simulink model "VCVS_lin_in_comm_out_comm"  (Simulink 7.5)
settings: Solver=ode45  StartTime=0.0  StopTime=10.0  RelTol=1e-3
settings Model: Creator=tugui_cat  LastModifiedBy=tugui
settings DebuggingCC: StrictBusMsg=Warning

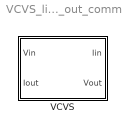
== system VCVS_lin_in_comm_out_comm ==
  VCVS : Subsystem  mask{Num_TF_dir1=1, Den_TF_dir1=1, Num_TF_inv1=1, Den_TF_inv1=1, Num_Zin1=1, Den_Zin1=1, Num_Zout1=1, Den_Zout1=1, OffIn11=0, OffIn12=0, OffOut11=0, OffOut12=0}
      mask help: Current-Controlled-Current-Source - linear model

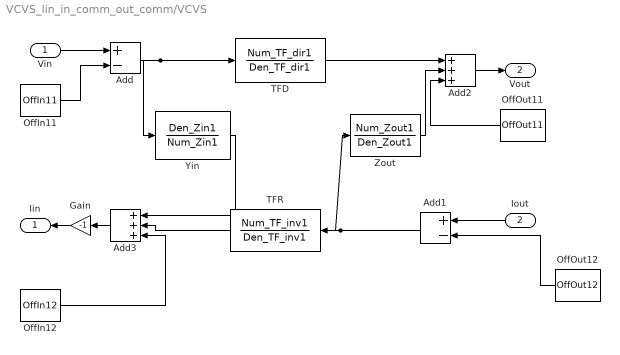
== system VCVS_lin_in_comm_out_comm/VCVS ==
  Vin : Inport
  Iout : Inport  Port=2
  Add : Sum  Inputs=+-  OutDataType=fixdt(1, 16)  OutScaling=2^-10
  Add1 : Sum  Inputs=+-  OutDataType=fixdt(1, 16)  OutScaling=2^-10
  Add2 : Sum  Inputs=+++  OutDataType=fixdt(1, 16)  OutScaling=2^-10
  Add3 : Sum  Inputs=+++  OutDataType=fixdt(1, 16)  OutScaling=2^-10
  Gain : Gain  Gain=-1  ParameterDataType=fixdt(1, 16)  ParameterScaling=2^0  OutDataType=fixdt(1, 16)  OutScaling=2^0
  OffIn11 : Constant  Value=OffIn11  OutDataType=fixdt(1, 16)  OutScaling=2^0
  OffIn12 : Constant  Value=OffIn12  OutDataType=fixdt(1, 16)  OutScaling=2^0
  OffOut11 : Constant  Value=OffOut11  OutDataType=fixdt(1, 16)  OutScaling=2^0
  OffOut12 : Constant  Value=OffOut12  OutDataType=fixdt(1, 16)  OutScaling=2^0
  TFD : TransferFcn  Numerator=Num_TF_dir1  Denominator=Den_TF_dir1
  TFR : TransferFcn  Numerator=Num_TF_inv1  Denominator=Den_TF_inv1
  Yin : TransferFcn  Numerator=Den_Zin1  Denominator=Num_Zin1
  Zout : TransferFcn  Numerator=Num_Zout1  Denominator=Den_Zout1
  Iin : Outport
  Vout : Outport  Port=2
  wires:
  Add2/1 -> Vout/1
  TFD/1 -> Add2/1
  Yin/1 -> Add3/1
  TFR/1 -> Add3/2
  Zout/1 -> Add2/2
  Vin/1 -> Add/1
  Add/1 -> Yin/1, TFD/1
  OffIn11/1 -> Add/2
  Iout/1 -> Add1/1
  Add1/1 -> Zout/1, TFR/1
  OffOut12/1 -> Add1/2
  OffIn12/1 -> Add3/3
  OffOut11/1 -> Add2/3
  Gain/1 -> Iin/1
  Add3/1 -> Gain/1
